simulink model "dynamic_approach_modeling"  (R2021a)
settings: Solver=VariableStepAuto  StartTime=0.0  StopTime=1100  MaxStep=0.1  RelTol=1e-3
values from neighbouring files (symbols this model uses):
  A_power = 30000    [powertrain_dynamic_approach_modeling.m]
  Area_V = 3.8056    [powertrain_dynamic_approach_modeling.m]
  B_f = 10000    [powertrain_dynamic_approach_modeling.m]
  B_Voltage = 364    [powertrain_dynamic_approach_modeling.m]
  Cd = 0.28    [powertrain_dynamic_approach_modeling.m]
  Crr = 0.015    [powertrain_dynamic_approach_modeling.m]
  D_mass = 80    [powertrain_dynamic_approach_modeling.m]
  G_R = 7.9    [powertrain_dynamic_approach_modeling.m]
  Mass_V = 1710.655    [powertrain_dynamic_approach_modeling.m]
  Motor_cont_efficiency = Motor_Cont(1:15,2:16)    [powertrain_dynamic_approach_modeling.m]
  Motor_cont_efficiency_regen = Motor_Cont_regen(1:15,2:16)    [powertrain_dynamic_approach_modeling.m]
  Motor_cont_speed = Motor_Cont(1:15,1)    [powertrain_dynamic_approach_modeling.m]
  Motor_cont_speed_regen = Motor_Cont_regen(1:15,1)    [powertrain_dynamic_approach_modeling.m]
  Motor_cont_torque = Motor_Cont(1:15,17)    [powertrain_dynamic_approach_modeling.m]
  Motor_cont_torque_regen = Motor_Cont_regen(1:15,17)    [powertrain_dynamic_approach_modeling.m]
  Motor_efficiency = Motor_eff(1:15,2:16)    [powertrain_dynamic_approach_modeling.m]
  Motor_efficiency_regen = Motor_eff_regen(1:15,2:16)    [powertrain_dynamic_approach_modeling.m]
  Motor_speed = Motor_eff(1:15,1)    [powertrain_dynamic_approach_modeling.m]
  Motor_speed_regen = Motor_eff_regen(1:15,1)    [powertrain_dynamic_approach_modeling.m]
  Motor_torque = Motor_eff(1:15,17)    [powertrain_dynamic_approach_modeling.m]
  Motor_torque_regen = Motor_eff_regen(1:15,17)    [powertrain_dynamic_approach_modeling.m]
  Rho = 1.225    [powertrain_dynamic_approach_modeling.m]
  Rw = 0.2032    [powertrain_dynamic_approach_modeling.m]
libraries: pid_lib x1
settings Model: Creator=LENOVO  LastModifiedBy=LENOVO

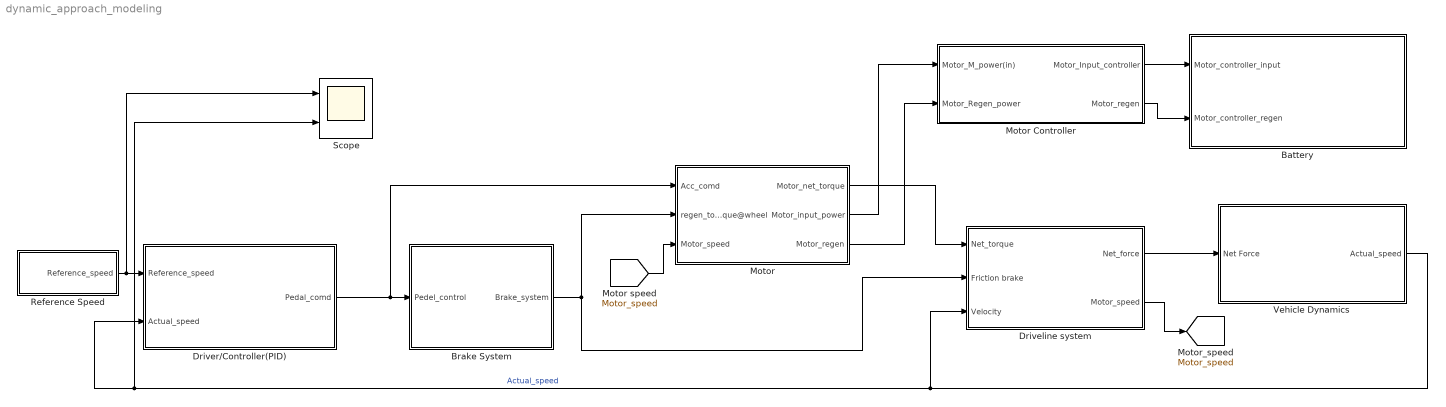
== system dynamic_approach_modeling ==
  Battery : Subsystem
  Brake System : Subsystem
  Driveline system : Subsystem
  Driver/Controller(PID) : Subsystem
  Motor : Subsystem
  Motor Controller : Subsystem
  Reference Speed : Subsystem
  Scope : Scope  NumInputPorts=2
  Vehicle Dynamics : Subsystem
  tag scope: Motor_speed=global
  wires:
  Vehicle Dynamics/1(Actual_speed) -> Driver/Controller(PID)/2(Actual_speed), Scope/2, Driveline system/3(Velocity)  "Actual_speed"
  Driver/Controller(PID)/1(Pedal_comd) -> Motor/1(Acc_comd), Brake System/1(Pedel_control)
  Brake System/1(Brake_system) -> Driveline system/2(Friction brake), Motor/2(regen_torque@wheel)
  Motor/1(Motor_net_torque) -> Driveline system/1(Net_torque)
  Driveline system/1(Net_force) -> Vehicle Dynamics/1(Net Force)
  Reference Speed/1(Reference_speed) -> Scope/1, Driver/Controller(PID)/1(Reference_speed)
  Driveline system/2(Motor_speed) -> [Motor_speed]
  [Motor_speed] -> Motor/3(Motor_speed)
  Motor/2(Motor_input_power) -> Motor Controller/1(Motor_M_power(in))
  Motor/3(Motor_regen) -> Motor Controller/2(Motor_Regen_power)
  Motor Controller/1(Motor_Input_controller) -> Battery/1(Motor_controller_input)
  Motor Controller/2(Motor_regen) -> Battery/2(Motor_controller_regen)

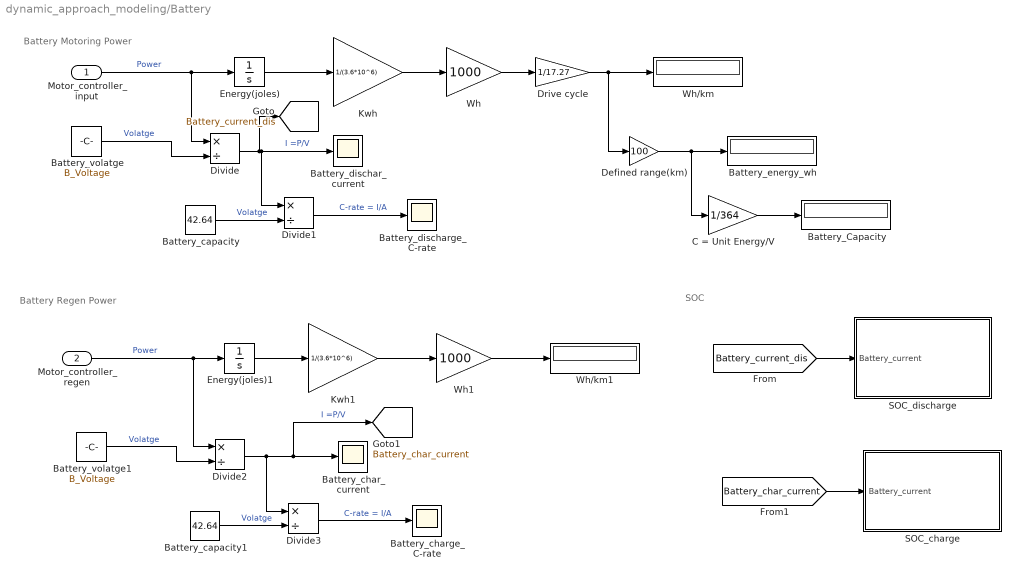
== system dynamic_approach_modeling/Battery ==
  note: SOC
  note: Battery Regen Power
  note: Battery Motoring Power
  Motor_controller_input : Inport
  Motor_controller_regen : Inport  Port=2
  Battery_Capacity : Display
  Battery_capacity : Constant  Value=42.64
  Battery_capacity1 : Constant  Value=42.64
  Battery_char_current : Scope
  Battery_charge_C-rate : Scope
  Battery_dischar_current : Scope
  Battery_discharge_C-rate : Scope
  Battery_energy_wh : Display
  Battery_volatge : Constant  Value=B_Voltage
  Battery_volatge1 : Constant  Value=B_Voltage
  C = Unit Energy/V : Gain  Gain=1/364
  Defined range(km) : Gain  Gain=100
  Divide{,1..3} (4 alike) : Product  Inputs=*/
  Drive cycle : Gain  Gain=1/17.27
  Energy(joles) : Integrator
  Energy(joles)1 : Integrator
  Kwh : Gain  Gain=1/(3.6*10^6)
  Kwh1 : Gain  Gain=1/(3.6*10^6)
  SOC_charge : Subsystem
  SOC_discharge : Subsystem
  Wh : Gain  Gain=1000
  Wh/km : Display
  Wh/km1 : Display
  Wh1 : Gain  Gain=1000
  tag scope: Battery_char_current=global, Battery_current_dis=global
  wires:
  Motor_controller_input/1 -> Energy(joles)/1, Divide/1  "Power"
  Battery_volatge/1 -> Divide/2  "Volatge"
  Divide/1 -> Battery_dischar_current/1, Divide1/1, [Battery_current_dis]  "I =P/V"
  Energy(joles)/1 -> Kwh/1
  Kwh/1 -> Wh/1
  Wh/1 -> Drive cycle/1
  Drive cycle/1 -> Defined range(km)/1, Wh/km/1
  Defined range(km)/1 -> C = Unit Energy/V/1, Battery_energy_wh/1
  C = Unit Energy/V/1 -> Battery_Capacity/1
  Battery_capacity/1 -> Divide1/2  "Volatge"
  Divide1/1 -> Battery_discharge_C-rate/1  "C-rate = I/A"
  Wh1/1 -> Wh/km1/1
  Energy(joles)1/1 -> Kwh1/1
  Kwh1/1 -> Wh1/1
  Divide2/1 -> Divide3/1, [Battery_char_current], Battery_char_current/1  "I =P/V"
  Divide3/1 -> Battery_charge_C-rate/1  "C-rate = I/A"
  Motor_controller_regen/1 -> Divide2/1, Energy(joles)1/1  "Power"
  Battery_capacity1/1 -> Divide3/2  "Volatge"
  Battery_volatge1/1 -> Divide2/2  "Volatge"
  [Battery_current_dis] -> SOC_discharge/1(Battery_current)
  [Battery_char_current] -> SOC_charge/1(Battery_current)

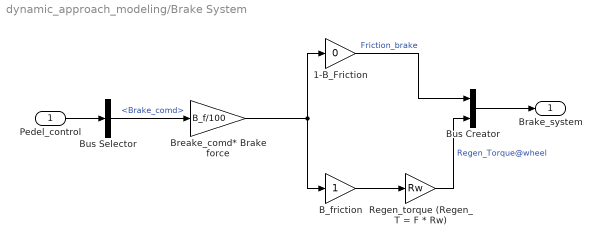
== system dynamic_approach_modeling/Brake System ==
  Pedel_control : Inport
  1-B_Friction : Gain  Gain=0
  B_friction : Gain
  Breake_comd* Brake force : Gain  Gain=B_f/100
  Bus Creator : BusCreator  Inputs=2
  Bus Selector : BusSelector  OutputSignals=Brake_comd
  Regen_torque (Regen_T = F * Rw) : Gain  Gain=Rw
  Brake_system : Outport
  wires:
  Pedel_control/1 -> Bus Selector/1
  Bus Selector/1 -> Breake_comd* Brake force/1  "<Brake_comd>"
  Breake_comd* Brake force/1 -> 1-B_Friction/1, B_friction/1
  B_friction/1 -> Regen_torque (Regen_T = F * Rw)/1
  1-B_Friction/1 -> Bus Creator/1  "Friction_brake"
  Regen_torque (Regen_T = F * Rw)/1 -> Bus Creator/2  "Regen_Torque@wheel"
  Bus Creator/1 -> Brake_system/1

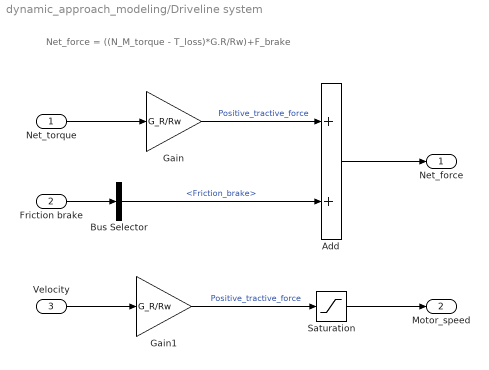
== system dynamic_approach_modeling/Driveline system ==
  note: Net_force = ((N_M_torque - T_loss)*G.R/Rw)+F_brake
  Net_torque : Inport
  Friction brake : Inport  Port=2
  Velocity : Inport  Port=3
  Add : Sum
  Bus Selector : BusSelector  OutputSignals=Friction_brake
  Gain : Gain  Gain=G_R/Rw
  Gain1 : Gain  Gain=G_R/Rw
  Saturation : Saturate  UpperLimit=inf  LowerLimit=0.00001
  Net_force : Outport
  Motor_speed : Outport  Port=2
  wires:
  Net_torque/1 -> Gain/1
  Gain/1 -> Add/1  "Positive_tractive_force"
  Friction brake/1 -> Bus Selector/1
  Bus Selector/1 -> Add/2  "<Friction_brake>"
  Velocity/1 -> Gain1/1
  Gain1/1 -> Saturation/1  "Positive_tractive_force"
  Add/1 -> Net_force/1
  Saturation/1 -> Motor_speed/1

== system dynamic_approach_modeling/Driver//Controller(PID) ==
  note: PID
  Reference_speed : Inport
  Actual_speed : Inport  Port=2
  Acceleration_comd : Saturate  UpperLimit=100  LowerLimit=0
  Brake_comd : Saturate  UpperLimit=0  LowerLimit=-100
  Bus Creator : BusCreator  Inputs=2
  Error_estimator : Sum  Inputs=+-
  PID Controller : pid_lib/PID Controller  Controller=PID  Form=Parallel  TimeDomain=Continuous-time  UseExternalTs=off  SampleTime=-1  IntegratorMethod=Forward Euler  FilterMethod=Forward Euler  ControllerParametersSource=internal  P=3000  I=3  D=1  UseFilter=on  N=100  TunerSelectOption=Transfer Function Based (PID Tuner App)  InitialConditionSource=internal  InitialConditionForIntegrator=0  InitialConditionForFilter=0  DifferentiatorICPrevScaledInput=0  ExternalReset=none  TrackingMode=off  Kt=1  LimitOutput=off  SatLimitsSource=internal  UpperSaturationLimit=inf  LowerSaturationLimit=-inf  LinearizeAsGain=on  AntiWindupMode=none  Kb=1  POutMin=[]  POutMax=[]  IOutMin=[]  IOutMax=[]  DOutMin=[]  DOutMax=[]  NOutMin=[]  NOutMax=[]  SumOutMin=[]  SumOutMax=[]  SaturationOutMin=[]  SaturationOutMax=[]  PParamMin=[]  PParamMax=[]  IParamMin=[]  IParamMax=[]  DParamMin=[]  DParamMax=[]  NParamMin=[]  NParamMax=[]  KbParamMin=[]  KbParamMax=[]  KtParamMin=[]  KtParamMax=[]  KbOutMin=[]  KbOutMax=[]  KtOutMin=[]  KtOutMax=[]  IntegratorOutMin=[]  IntegratorOutMax=[]  FilterOutMin=[]  FilterOutMax=[]  SumI1OutMin=[]  SumI1OutMax=[]  SumI2OutMin=[]  SumI2OutMax=[]  SumI3OutMin=[]  SumI3OutMax=[]  SumI4OutMin=[]  SumI4OutMax=[]  SumDOutMin=[]  SumDOutMax=[]  DifferentiatorOutMin=[]  DifferentiatorOutMax=[]  FilterDiffOutCoefMin=[]  FilterDiffOutCoefMax=[]  ReciprocalOutMin=[]  ReciprocalOutMax=[]  SumDenOutMin=[]  SumDenOutMax=[]  SumNumOutMin=[]  SumNumOutMax=[]  DivideOutMin=[]  DivideOutMax=[]  UdiffTsProdOutMin=[]  UdiffTsProdOutMax=[]  NTsProdOutMin=[]  NTsProdOutMax=[]  UintegralTsProdOutMin=[]  UintegralTsProdOutMax=[]  UngainTsProdOutMin=[]  UngainTsProdOutMax=[]  IntegratorContinuousStateAttributes=''  IntegratorStateMustResolveToSignalObject=off  IntegratorRTWStateStorageClass=Auto  FilterContinuousStateAttributes=''  FilterStateMustResolveToSignalObject=off  FilterRTWStateStorageClass=Auto  ParallelPVariant=InternalParameters  IdealPVariant=Disabled  IVariant=InternalParameters  DVariant=InternalParameters  IntegratorVariant=Continuous  SatVariant=Disabled  AWVariant=Passthrough  PCopyVariant=Disabled  TRVariant=Disabled  FdbkBlocksVariant=Forward  IdealPFdbkVariant=Disabled  SatFdbkVariant=Disabled  DerivativeFilterVariant=ContFilter  NVariant=InternalParameters  NCopyVariant=Disabled  FilterICVariant=InternalICsFilter  IntegratorICVariant=InternalICs  ExternalResetVariant=Disabled  TRSumVariant=Passthrough  SumFdbkVariant=Disabled  SumVariant=Sum_PID  TsampFilterVariant=InternalTs  TsampNgainVariant=Passthrough  TsampIntegralVariant=Passthrough  ExternalSaturationOutDataTypeStr=Inherit: Same as second input
  Pedal_comd : Outport
  wires:
  Reference_speed/1 -> Error_estimator/1
  Actual_speed/1 -> Error_estimator/2
  Error_estimator/1 -> PID Controller/1
  PID Controller/1 -> Brake_comd/1, Acceleration_comd/1
  Acceleration_comd/1 -> Bus Creator/1  "Acc_comd"
  Brake_comd/1 -> Bus Creator/2  "Brake_comd"
  Bus Creator/1 -> Pedal_comd/1

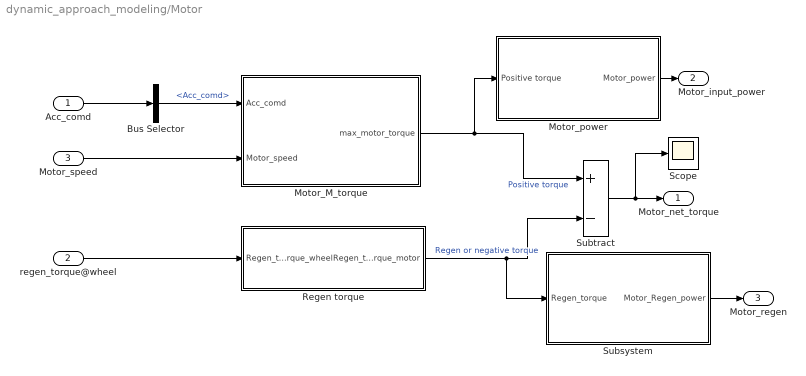
== system dynamic_approach_modeling/Motor ==
  Acc_comd : Inport
  regen_torque@wheel : Inport  Port=2
  Motor_speed : Inport  Port=3
  Bus Selector : BusSelector  OutputSignals=Acc_comd
  Motor_M_torque : Subsystem
  Motor_power : Subsystem
  Regen torque : Subsystem
  Scope : Scope
  Subsystem : Subsystem
  Subtract : Sum  Inputs=+-
  Motor_net_torque : Outport
  Motor_input_power : Outport  Port=2
  Motor_regen : Outport  Port=3
  wires:
  Acc_comd/1 -> Bus Selector/1
  regen_torque@wheel/1 -> Regen torque/1(Regen_torque_wheel)
  Bus Selector/1 -> Motor_M_torque/1(Acc_comd)  "<Acc_comd>"
  Motor_speed/1 -> Motor_M_torque/2(Motor_speed)
  Motor_M_torque/1(max_motor_torque) -> Subtract/1, Motor_power/1(Positive torque)  "Positive torque"
  Regen torque/1(Regen_torque_motor) -> Subsystem/1(Regen_torque), Subtract/2  "Regen or negative torque"
  Subtract/1 -> Scope/1, Motor_net_torque/1
  Motor_power/1(Motor_power) -> Motor_input_power/1
  Subsystem/1(Motor_Regen_power) -> Motor_regen/1

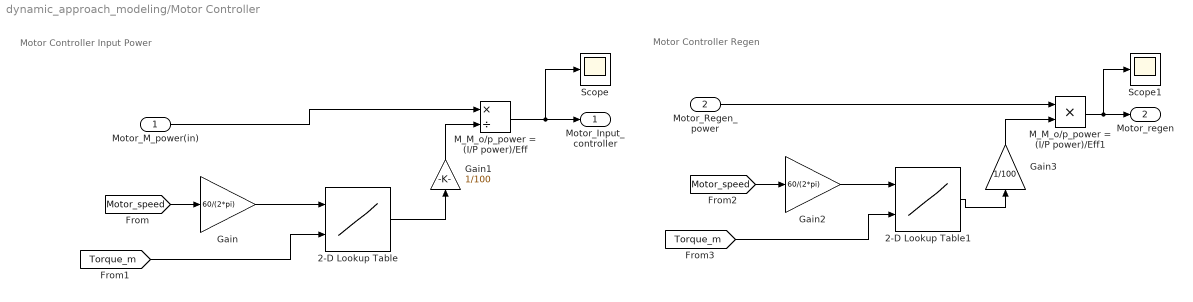
== system dynamic_approach_modeling/Motor Controller ==
  note: Motor Controller Regen
  note: Motor Controller Input Power
  Motor_M_power(in) : Inport
  Motor_Regen_power : Inport  Port=2
  2-D Lookup Table : Lookup_n-D  BreakpointsForDimension1=Motor_cont_speed  BreakpointsForDimension2=Motor_cont_torque  Table=Motor_cont_efficiency  InternalRulePriority=Speed  RndMeth=Simplest  InputSameDT=on
      settings: InputPortMap=u0,u1
  2-D Lookup Table1 : Lookup_n-D  BreakpointsForDimension1=Motor_cont_speed_regen  BreakpointsForDimension2=Motor_cont_torque_regen  Table=Motor_cont_efficiency_regen  InternalRulePriority=Speed  RndMeth=Simplest  InputSameDT=on
      settings: InputPortMap=u0,u1
  Gain : Gain  Gain=60/(2*pi)
  Gain1 : Gain  Gain=1/100
  Gain2 : Gain  Gain=60/(2*pi)
  Gain3 : Gain  Gain=1/100
  M_M_o/p_power = (I/P power)/Eff : Product  Inputs=*/
  M_M_o/p_power = (I/P power)/Eff1 : Product  Inputs=**
  Scope : Scope
  Scope1 : Scope
  Motor_Input_controller : Outport
  Motor_regen : Outport  Port=2
  wires:
  [Motor_speed] -> Gain/1
  Gain/1 -> 2-D Lookup Table/1
  [Torque_m] -> 2-D Lookup Table/2
  2-D Lookup Table/1 -> Gain1/1
  Gain1/1 -> M_M_o/p_power = (I/P power)/Eff/2
  Motor_M_power(in)/1 -> M_M_o/p_power = (I/P power)/Eff/1
  M_M_o/p_power = (I/P power)/Eff/1 -> Scope/1, Motor_Input_controller/1
  [Torque_m] -> 2-D Lookup Table1/2
  2-D Lookup Table1/1 -> Gain3/1
  [Motor_speed] -> Gain2/1
  Gain2/1 -> 2-D Lookup Table1/1
  Motor_Regen_power/1 -> M_M_o/p_power = (I/P power)/Eff1/1
  Gain3/1 -> M_M_o/p_power = (I/P power)/Eff1/2
  M_M_o/p_power = (I/P power)/Eff1/1 -> Motor_regen/1, Scope1/1

== system dynamic_approach_modeling/Reference Speed ==
  Gain : Gain  Gain=1000/3600
  Multiport Switch : MultiPortSwitch  Inputs=4
  NEDC_Drive Cycle : FromWorkspace  VariableName=data
  Rural_Drive_Cycle : FromWorkspace  VariableName=data2
  Speed_profile_1 : Constant  Value=100
  Speed_selector : Constant  Value=4
  Urban_Drive_Cycle : FromWorkspace  VariableName=data1
  Reference_speed : Outport
  wires:
  Speed_selector/1 -> Multiport Switch/1
  Speed_profile_1/1 -> Multiport Switch/2
  NEDC_Drive Cycle/1 -> Multiport Switch/3
  Multiport Switch/1 -> Gain/1
  Gain/1 -> Reference_speed/1
  Urban_Drive_Cycle/1 -> Multiport Switch/4
  Rural_Drive_Cycle/1 -> Multiport Switch/5

== system dynamic_approach_modeling/Vehicle Dynamics ==
  note: Actual Speed
  note: F_acc = Net force - F_Aero-F_gradient_F_Rolling
  Net Force : Inport
  Aerodynamic Force : Subsystem
  Gain : Gain  Gain=1/(D_mass+Mass_V)
  Gradient Force : Subsystem
  Integrator : Integrator
  Rolling force : Subsystem
  Subtract : Sum  Inputs=+---
  Actual_speed : Outport
  wires:
  Net Force/1 -> Subtract/1
  Rolling force/1(Rolling_force) -> Subtract/2
  Gradient Force/1(Gradient_force) -> Subtract/3
  Aerodynamic Force/1(Aerodynamic_force) -> Subtract/4
  Gain/1 -> Integrator/1  "F=M*a (N) Acc= Force/Mass(m/s^2)"
  Integrator/1 -> Aerodynamic Force/1(Velocity), Actual_speed/1  "m/s"
  Subtract/1 -> Gain/1  "F(N)"

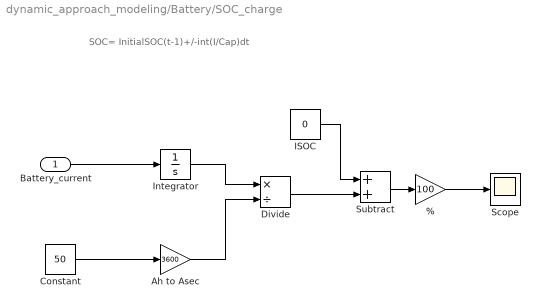
== system dynamic_approach_modeling/Battery/SOC_charge ==
  note: SOC= InitialSOC(t-1)+/-int(I/Cap)dt
  Battery_current : Inport
  % : Gain  Gain=100
  Ah to Asec : Gain  Gain=3600
  Constant : Constant  Value=50
  Divide : Product  Inputs=*/
  ISOC : Constant  Value=0
  Integrator : Integrator
  Scope : Scope
  Subtract : Sum
  wires:
  Battery_current/1 -> Integrator/1
  Constant/1 -> Ah to Asec/1
  Integrator/1 -> Divide/1
  Ah to Asec/1 -> Divide/2
  Divide/1 -> Subtract/2
  ISOC/1 -> Subtract/1
  Subtract/1 -> %/1
  %/1 -> Scope/1

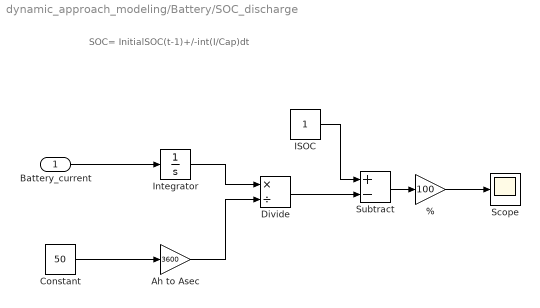
== system dynamic_approach_modeling/Battery/SOC_discharge ==
  note: SOC= InitialSOC(t-1)+/-int(I/Cap)dt
  Battery_current : Inport
  % : Gain  Gain=100
  Ah to Asec : Gain  Gain=3600
  Constant : Constant  Value=50
  Divide : Product  Inputs=*/
  ISOC : Constant
  Integrator : Integrator
  Scope : Scope
  Subtract : Sum  Inputs=+-
  wires:
  Battery_current/1 -> Integrator/1
  Constant/1 -> Ah to Asec/1
  Integrator/1 -> Divide/1
  Ah to Asec/1 -> Divide/2
  Divide/1 -> Subtract/2
  ISOC/1 -> Subtract/1
  Subtract/1 -> %/1
  %/1 -> Scope/1

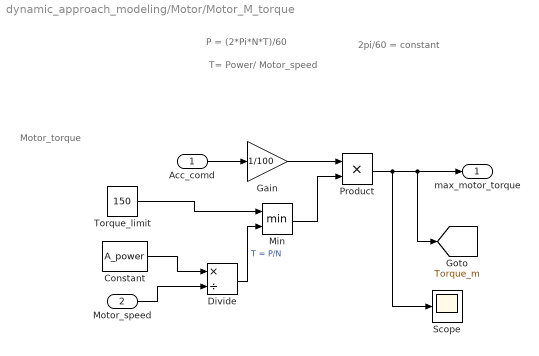
== system dynamic_approach_modeling/Motor/Motor_M_torque ==
  note: Motor_torque
  note: T= Power/ Motor_speed
  note: 2pi/60 = constant
  note: P = (2*Pi*N*T)/60
  Acc_comd : Inport
  Motor_speed : Inport  Port=2
  Constant : Constant  Value=A_power
  Divide : Product  Inputs=*/
  Gain : Gain  Gain=1/100
  Min : MinMax  Inputs=2
  Product : Product
  Scope : Scope
  Torque_limit : Constant  Value=150
  max_motor_torque : Outport
  tag scope: Torque_m=global
  wires:
  Acc_comd/1 -> Gain/1
  Gain/1 -> Product/1
  Constant/1 -> Divide/1
  Motor_speed/1 -> Divide/2
  Torque_limit/1 -> Min/1
  Divide/1 -> Min/2  "T = P/N"
  Min/1 -> Product/2
  Product/1 -> Scope/1, [Torque_m], max_motor_torque/1

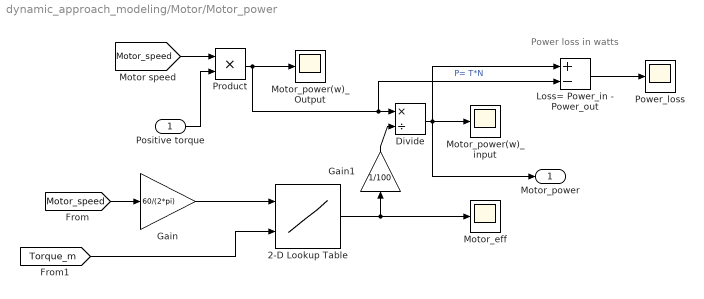
== system dynamic_approach_modeling/Motor/Motor_power ==
  note: Power loss in watts
  Positive torque : Inport
  2-D Lookup Table : Lookup_n-D  BreakpointsForDimension1=Motor_speed  BreakpointsForDimension2=Motor_torque  Table=Motor_efficiency  InternalRulePriority=Speed  RndMeth=Simplest  InputSameDT=on
      settings: InputPortMap=u0,u1
  Divide : Product  Inputs=*/
  Gain : Gain  Gain=60/(2*pi)
  Gain1 : Gain  Gain=1/100
  Loss= Power_in - Power_out : Sum  Inputs=+-
  Motor_eff : Scope
  Motor_power(w)_Output : Scope
  Motor_power(w)_input : Scope
  Power_loss : Scope
  Product : Product
  Motor_power : Outport
  wires:
  [Motor_speed] -> Product/1
  Product/1 -> Motor_power(w)_Output/1, Loss= Power_in - Power_out/2, Divide/1  "P= T*N"
  Positive torque/1 -> Product/2
  [Motor_speed] -> Gain/1
  2-D Lookup Table/1 -> Motor_eff/1, Gain1/1
  Gain1/1 -> Divide/2
  Divide/1 -> Motor_power/1, Loss= Power_in - Power_out/1, Motor_power(w)_input/1
  Gain/1 -> 2-D Lookup Table/1
  [Torque_m] -> 2-D Lookup Table/2
  Loss= Power_in - Power_out/1 -> Power_loss/1

== system dynamic_approach_modeling/Motor/Regen torque ==
  note: Regen torque
  note: Torque = (Force*Radius_wheel)/G.R
  Regen_torque_wheel : Inport
  Abs : Abs
  Regen_motor_torque = Regen_wheel_torque/GR : Gain  Gain=1/G_R
  Regen_torque : BusSelector  OutputSignals=Regen_Torque@wheel
  Regen_torque_motor : Outport
  wires:
  Regen_torque/1 -> Regen_motor_torque = Regen_wheel_torque/GR/1  "<Regen_Torque@wheel>"
  Regen_motor_torque = Regen_wheel_torque/GR/1 -> Abs/1
  Abs/1 -> Regen_torque_motor/1
  Regen_torque_wheel/1 -> Regen_torque/1

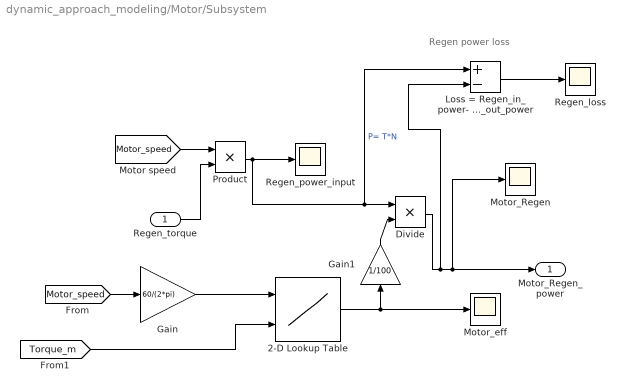
== system dynamic_approach_modeling/Motor/Subsystem ==
  note: Regen power loss
  Regen_torque : Inport
  2-D Lookup Table : Lookup_n-D  BreakpointsForDimension1=Motor_speed_regen  BreakpointsForDimension2=Motor_torque_regen  Table=Motor_efficiency_regen  InternalRulePriority=Speed  RndMeth=Simplest  InputSameDT=on
      settings: InputPortMap=u0,u1
  Divide : Product  Inputs=**
  Gain : Gain  Gain=60/(2*pi)
  Gain1 : Gain  Gain=1/100
  Loss = Regen_in_power- Regen_out_power : Sum  Inputs=+-
  Motor_Regen : Scope
  Motor_eff : Scope
  Product : Product
  Regen_loss : Scope
  Regen_power_input : Scope
  Motor_Regen_power : Outport
  wires:
  Divide/1 -> Loss = Regen_in_power- Regen_out_power/2, Motor_Regen_power/1, Motor_Regen/1
  Gain/1 -> 2-D Lookup Table/1
  [Torque_m] -> 2-D Lookup Table/2
  Regen_torque/1 -> Product/2
  [Motor_speed] -> Gain/1
  Product/1 -> Regen_power_input/1, Loss = Regen_in_power- Regen_out_power/1, Divide/1  "P= T*N"
  Gain1/1 -> Divide/2
  2-D Lookup Table/1 -> Motor_eff/1, Gain1/1
  [Motor_speed] -> Product/1
  Loss = Regen_in_power- Regen_out_power/1 -> Regen_loss/1

== system dynamic_approach_modeling/Vehicle Dynamics/Aerodynamic Force ==
  note: Aerodynamic force
  note: F_Aero = 0.5*Cdd*F_a*Rho*V^2
  Velocity : Inport
  Air density : Constant  Value=Rho
  Constant : Constant  Value=0.5
  Frontal Area : Constant  Value=Area_V
  Product : Product  Inputs=5
  Square : Math  Operator=square  SaturateOnIntegerOverflow=on
  coefficient of drag : Constant  Value=Cd
  Aerodynamic_force : Outport
  wires:
  Velocity/1 -> Square/1
  Constant/1 -> Product/1
  coefficient of drag/1 -> Product/2
  Air density/1 -> Product/3
  Frontal Area/1 -> Product/4
  Square/1 -> Product/5
  Product/1 -> Aerodynamic_force/1

== system dynamic_approach_modeling/Vehicle Dynamics/Gradient Force ==
  note: Gradient
      | force
  note: F_grad = GVW*Sin(theta)
  Gain : Gain  Gain=sin(0)
  Gradient_force : Outport
  wires:
  [GVM] -> Gain/1
  Gain/1 -> Gradient_force/1

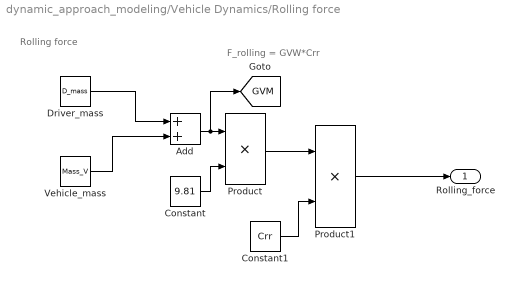
== system dynamic_approach_modeling/Vehicle Dynamics/Rolling force ==
  note: Rolling force
  note: F_rolling = GVW*Crr
  Add : Sum
  Constant : Constant  Value=9.81
  Constant1 : Constant  Value=Crr
  Driver_mass : Constant  Value=D_mass
  Product : Product
  Product1 : Product
  Vehicle_mass : Constant  Value=Mass_V
  Rolling_force : Outport
  tag scope: GVM=global
  wires:
  Driver_mass/1 -> Add/1
  Vehicle_mass/1 -> Add/2
  Add/1 -> [GVM], Product/1
  Constant/1 -> Product/2
  Product/1 -> Product1/1
  Constant1/1 -> Product1/2
  Product1/1 -> Rolling_force/1
